simulink model "Week3_LOC4_deel2_v2_1"  (R2021b)
settings: Solver=FixedStepDiscrete  StartTime=0.0  StopTime=inf  RelTol=1e-3
libraries: arduinolib x8
settings Model: FPTRunName=Active  ExtModeTrigDuration=2  Creator=889450  LastModifiedBy=Jeedella
settings SolverCC: AlgebraicLoopSolver=TrustRegion
settings DataIOCC: LimitDataPoints=on  SaveFormat=Array
settings OptimizationCC: ExpressionDepthLimit=2147483647  LifeSpan=Inf  MaxStackSize=64
settings DebuggingCC: UnderspecifiedInitializationDetection=Classic  MergeDetectMultiDrivingBlocksExec=none  FcnCallInpInsideContextMsg=warning  AllowSymbolicDim=off  StateNameClashWarn=warning  SFUnexpectedBacktrackingDiag=warning  SFNoUnconditionalDefaultTransitionDiag=warning  SFExecutionAtInitializationDiag=none  SFMachineParentedDataDiag=warning  ArithmeticOperatorsInVariantConditions=warning
settings HardwareCC: ProdBitPerInt=16  ProdBitPerPointer=16  ProdBitPerSizeT=16  ProdBitPerPtrDiffT=16  ProdLargestAtomicFloat=None  ProdWordSize=8  ProdHWDeviceType=Atmel->AVR
settings ModelReferenceCC: PropagateSignalLabelsOutOfModel=off
settings SFSimCC: SimUseLocalCustomCode=off  CustomCodeUndefinedFunction=UseInterfaceOnly
settings RTWCC: Description=Embedded Coder  SystemTargetFile=ert.tlc  HardwareBoard=Arduino Uno  TemplateMakefile=ert_default_tmf  GenerateReport=on  RTWVerbose=off  RTWUseLocalCustomCode=off  Toolchain=Arduino AVR  BuildConfiguration=Faster Runs  LaunchReport=on
settings CodeAppCC: ForceParamTrailComments=on  OperatorAnnotations=on  StateflowObjectComments=on  MATLABSourceComments=on
settings ERTTargetCC: MultiwordLength=2048  ERTCustomFileBanners=off  SupportContinuousTime=on  SupportNonInlinedSFcns=on  RemoveResetFunc=off  SupportVariableSizeSignals=on  ModelStepFunctionPrototypeControlCompliant=off  ExtModeStaticAllocSize=250
settings ConfigComp: CovMetricSettings=dw  CovSaveCumulativeToWorkspaceVar=on  CovSaveSingleToWorkspaceVar=on  CovExternalEMLEnable=off  CovSFcnEnable=off

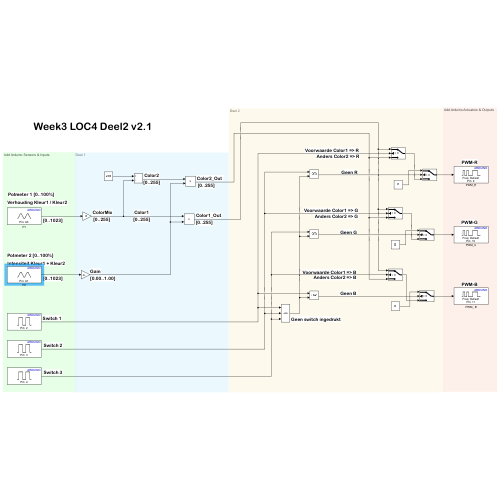
[thumbnail: Simulink's stored preview of the top-level diagram]
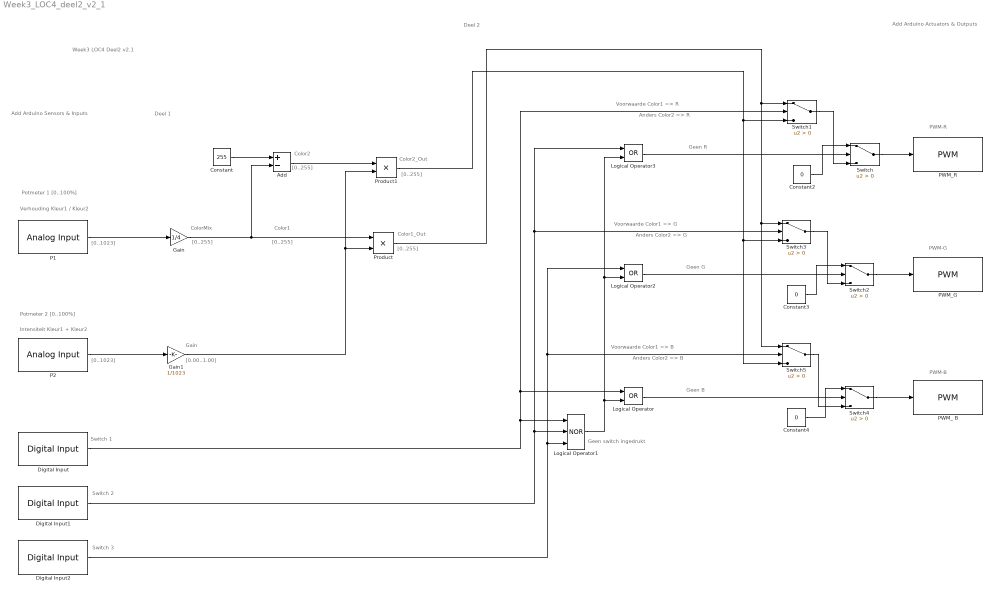
== system Week3_LOC4_deel2_v2_1 ==
  note: Week3 LOC4 Deel2 v2.1
  note: Potmeter 1 [0..100%]
  note: Potmeter 2 [0..100%]
  note: Verhouding Kleur1 / Kleur2
  note: Intensiteit Kleur1 + Kleur2
  note: [0..1023]
  note: [0..1023]
  note: [0..255]
  note: [0.00..1.00]
  note: Gain
  note: [0..255]
  note: Color1_Out
  note: Color2_Out
  note: PWM-R
  note: PWM-G
  note: PWM-B
  note: Add Arduino Sensors & Inputs
  note: Add Arduino Actuators & Outputs
  note: Deel 1
  note: ColorMix
  note: Color1
  note: [0..255]
  note: [0..255]
  note: Color2
  note: [0..255]
  note: Deel 2
  note: Anders Color2 => B
  note: Geen G
  note: Voorwaarde Color1 => G
  note: Anders Color2 => R
  note: Geen R
  note: Voorwaarde Color1 => B
  note: Geen B
  note: Geen switch ingedrukt
  note: Anders Color2 => G
  note: Voorwaarde Color1 => R
  note: Switch 1
  note: Switch 3
  note: Switch 2
  Add : Sum  Inputs=+-
  Constant : Constant  Value=255  SampleTime=-1
  Constant2 : Constant  Value=0  SampleTime=-1
  Constant3 : Constant  Value=0  SampleTime=-1
  Constant4 : Constant  Value=0  SampleTime=-1
  Digital Input : arduinolib/Digital Input  pinNumber=2  mode=Default  Direction=input  SampleTime=0.1  blockPlatform=arduino
  Digital Input1 : arduinolib/Digital Input  pinNumber=3  mode=Default  Direction=input  SampleTime=0.1  blockPlatform=arduino
  Digital Input2 : arduinolib/Digital Input  pinNumber=4  mode=Default  Direction=input  SampleTime=0.1  blockPlatform=arduino
  Gain : Gain  Gain=1/4
  Gain1 : Gain  Gain=1/1023
  Logical Operator : Logic  Operator=OR  AllPortsSameDT=off  OutDataTypeStr=boolean
  Logical Operator1 : Logic  Operator=NOR  Inputs=3  AllPortsSameDT=off  OutDataTypeStr=boolean
  Logical Operator2 : Logic  Operator=OR  AllPortsSameDT=off  OutDataTypeStr=boolean
  Logical Operator3 : Logic  Operator=OR  AllPortsSameDT=off  OutDataTypeStr=boolean
  P1 : arduinolib/Analog Input  pinNumber=0  ReadResultsOnly=off  ConversionTriggerSource=Software  ExternalTriggerType=uint32( 0 )  OutputDataType=uint16  EnableConversionCompleteNotify=off  EnableOuputStatus=off  SampleTime=-1  blockPlatform=arduino
  P2 : arduinolib/Analog Input  pinNumber=1  ReadResultsOnly=off  ConversionTriggerSource=Software  ExternalTriggerType=uint32( 0 )  OutputDataType=uint16  EnableConversionCompleteNotify=off  EnableOuputStatus=off  SampleTime=-1  blockPlatform=arduino
  PWM_ B : arduinolib/PWM  pinNumber=11  frequencyType=Default  desiredFrequency=490.2  achievableFrequency=490.2
  PWM_G : arduinolib/PWM  pinNumber=10  frequencyType=Default  desiredFrequency=490.2  achievableFrequency=490.2
  PWM_R : arduinolib/PWM  pinNumber=9  frequencyType=Default  desiredFrequency=490.2  achievableFrequency=490.2
  Product : Product
  Product1 : Product
  Switch{,1..5} (6 alike) : Switch  Criteria=u2 > Threshold
  wires:
  P1/1 -> Gain/1
  Gain/1 -> Add/2, Product/1
  Add/1 -> Product1/1
  Constant/1 -> Add/1
  P2/1 -> Gain1/1
  Gain1/1 -> Product1/2, Product/2
  Logical Operator3/1 -> Switch/2
  Constant3/1 -> Switch2/1
  Logical Operator1/1 -> Logical Operator/2, Logical Operator3/2, Logical Operator2/2
  Product1/1 -> Switch5/3, Switch3/3, Switch1/3
  Constant2/1 -> Switch/1
  Digital Input2/1 -> Logical Operator1/3, Logical Operator2/1, Switch5/2
  Logical Operator/1 -> Switch4/2
  Product/1 -> Switch5/1, Switch3/1, Switch1/1
  Digital Input1/1 -> Logical Operator3/1, Switch3/2, Logical Operator1/2
  Constant4/1 -> Switch4/1
  Digital Input/1 -> Logical Operator1/1, Logical Operator/1, Switch1/2
  Switch1/1 -> Switch/3
  Switch5/1 -> Switch4/3
  Switch3/1 -> Switch2/3
  Logical Operator2/1 -> Switch2/2
  Switch/1 -> PWM_R/1
  Switch2/1 -> PWM_G/1
  Switch4/1 -> PWM_ B/1
